simulink model "Model_of_plantarflexions"  (R2019a)
settings: Solver=ode23s  StartTime=0  StopTime=60  FixedStep=0.001  MaxStep=0.1  RelTol=1e-4  EnableMultiTasking=on
values from neighbouring files (symbols this model uses):
  ankle_angle_60sec = deg2rad(ankle_angle_60sec)    [init_muscle_exp.m]
  MP = muscle_param_GM_exp    [init_muscle_exp.m]
undefined symbols (not defined in the file or in its folder): gm_norm_MVC, time
libraries: library_mtu_simulink x2
settings Model: NumberOfSteps=200  Creator=danielhaeufle  LastModifiedBy=danielhaeufle
settings SolverCC: ZeroCrossAlgorithm=Adaptive
settings DataIOCC: ReturnWorkspaceOutputs=off  OutputSaveName=Output
settings OptimizationCC: LifeSpan=inf
settings DebuggingCC: MaxConsecutiveZCsMsg=none  MaskedZcDiagnostic=none  IgnoredZcDiagnostic=none  PregeneratedLibrarySubsystemCodeDiagnostic=none  SFUnexpectedBacktrackingDiag=warning  SFNoUnconditionalDefaultTransitionDiag=warning  SFExecutionAtInitializationDiag=none  ArithmeticOperatorsInVariantConditions=warning
settings SFSimCC: SimUseLocalCustomCode=off
settings RTWCC: RTWUseLocalCustomCode=off
settings CodeAppCC: StateflowObjectComments=on
settings GRTTargetCC: TargetLangStandard=C89/C90 (ANSI)  GeneratePreprocessorConditionals=Disable all
settings ConfigComp: CovMetricSettings=dw  CovHtmlReporting=on  CovSaveCumulativeToWorkspaceVar=on  CovSaveSingleToWorkspaceVar=on  CovExternalEMLEnable=off

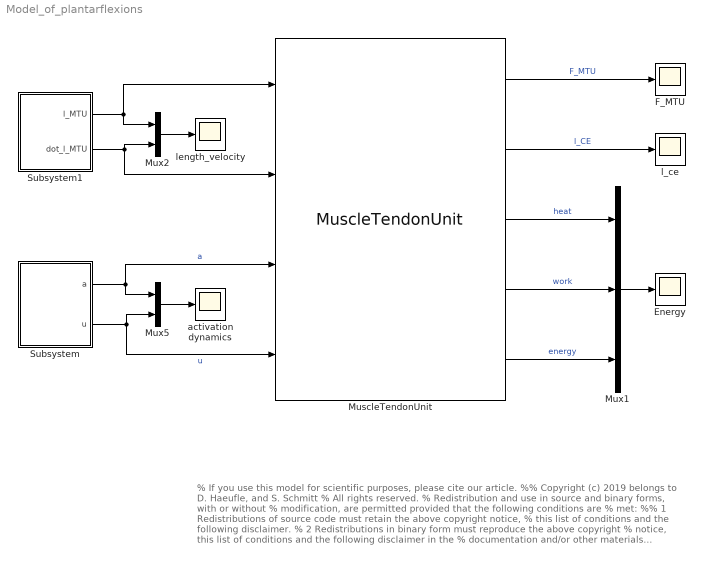
== system Model_of_plantarflexions ==
  note: % If you use this model for scientific purposes, please cite our article.
      | %% Copyright (c) 2019 belongs to D. Haeufle, and S. Schmitt % All rights reserved.
      | % Redistribution and use in source and binary forms, with or without
      | % modification, are permitted provided that the following conditions are
      | % met:
      | %%  1 Redistributions of source code must retain the above copyright notice,
      | %    this list of conditions and the following disclaimer.
      | %  2 Redistributions in binary form must reproduce the above copyright
      | %    notice, this list of conditions and the following disclaimer in the
      | %    documentation and/or other materials provided with the distribution.
      | %  3 Neither the name of the owner nor the names of its contributors may be
      | %    used to endorse or promote products derived from this software without
      | %    specific prior written permission.
      | %% THIS SOFTWARE IS PROVIDED BY THE COPYRIGHT HOLDERS AND CONTRIBUTORS "AS
      | % IS" AND ANY EXPRESS OR IMPLIED WARRANTIES, INCLUDING, BUT NOT LIMITED TO,
      | % THE IMPLIED WARRANTIES OF MERCHANTABILITY AND FITNESS FOR A PARTICULAR
      | % PURPOSE ARE DISCLAIMED. IN NO EVENT SHALL THE COPYRIGHT HOLDER BE LIABLE
      | % FOR ANY DIRECT, INDIRECT, INCIDENTAL, SPECIAL, EXEMPLARY, OR
      | % CONSEQUENTIAL DAMAGES (INCLUDING, BUT NOT LIMITED TO, PROCUREMENT OF
      | % SUBSTITUTE GOODS OR SERVICES; LOSS OF USE, DATA, OR PROFITS; OR BUSINESS
      | % INTERRUPTION) HOWEVER CAUSED AND ON ANY THEORY OF LIABILITY, WHETHER IN
      | % CONTRACT, STRICT LIABILITY, OR TORT (INCLUDING NEGLIGENCE OR OTHERWISE)
      | % ARISING IN ANY WAY OUT OF THE USE OF THIS SOFTWARE, EVEN IF ADVISED OF
      | % THE POSSIBILITY OF SUCH DAMAGE.
  Energy : Scope
  F_MTU : Scope
  MuscleTendonUnit : library_mtu_simulink/MuscleTendonUnit  Mus_Param=MP(1)
  Mux1 : Mux  Inputs=3
  Mux2 : Mux  Inputs=2
  Mux5 : Mux  Inputs=2
  Subsystem : Subsystem
  Subsystem1 : Subsystem
  activation dynamics : Scope
  l_ce : Scope
  length_velocity : Scope
  wires:
  Mux5/1 -> activation dynamics/1
  Mux1/1 -> Energy/1
  Subsystem1/2(dot_l_MTU) -> MuscleTendonUnit/2, Mux2/2
  Subsystem/1(a) -> MuscleTendonUnit/3, Mux5/1  "a"
  Subsystem/2(u) -> MuscleTendonUnit/4, Mux5/2  "u"
  MuscleTendonUnit/2 -> l_ce/1  "l_CE"
  MuscleTendonUnit/1 -> F_MTU/1  "F_MTU"
  MuscleTendonUnit/5 -> Mux1/3  "energy"
  MuscleTendonUnit/4 -> Mux1/2  "work"
  MuscleTendonUnit/3 -> Mux1/1  "heat"
  Mux2/1 -> length_velocity/1
  Subsystem1/1(l_MTU) -> MuscleTendonUnit/1, Mux2/1

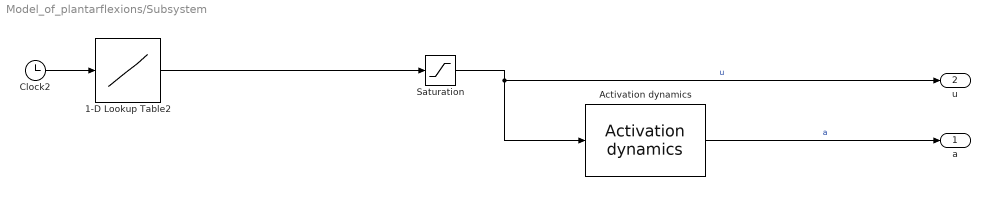
== system Model_of_plantarflexions/Subsystem ==
  1-D Lookup Table2 : Lookup_n-D  NumberOfTableDimensions=1  BreakpointsForDimension1=time  Table=gm_norm_MVC  InternalRulePriority=Speed  RndMeth=Simplest  InputSameDT=on
  Activation dynamics : library_mtu_simulink/Activation dynamics  Mus_Param=MP
  Clock2 : Clock
      settings: Decimation=100
  Saturation : Saturate  UpperLimit=1  LowerLimit=0.001
  a : Outport
  u : Outport  Port=2
  wires:
  Activation dynamics/1 -> a/1  "a"
  Saturation/1 -> u/1, Activation dynamics/1  "u"
  1-D Lookup Table2/1 -> Saturation/1
  Clock2/1 -> 1-D Lookup Table2/1

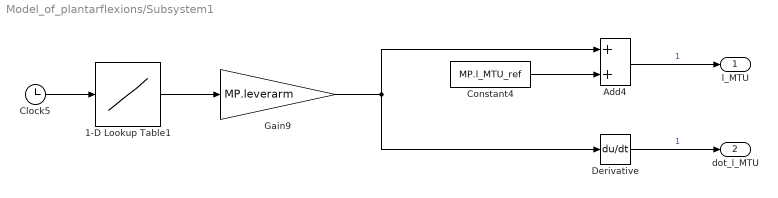
== system Model_of_plantarflexions/Subsystem1 ==
  1-D Lookup Table1 : Lookup_n-D  NumberOfTableDimensions=1  BreakpointsForDimension1=time  Table=ankle_angle_60sec  InternalRulePriority=Speed  RndMeth=Simplest  InputSameDT=on
  Add4 : Sum
  Clock5 : Clock
  Constant4 : Constant  Value=MP.l_MTU_ref
  Derivative : Derivative
  Gain9 : Gain  Gain=MP.leverarm
  l_MTU : Outport
  dot_l_MTU : Outport  Port=2
  wires:
  Constant4/1 -> Add4/2
  Gain9/1 -> Derivative/1, Add4/1
  1-D Lookup Table1/1 -> Gain9/1
  Derivative/1 -> dot_l_MTU/1  "1"
  Add4/1 -> l_MTU/1  "1"
  Clock5/1 -> 1-D Lookup Table1/1
